simulink model "EjemploClienteConNovint"  (Simulink 7.8)
settings: Solver=ode3  StartTime=0.0  StopTime=inf  FixedStep=0.001  RelTol=1e-3
libraries: aerolibanimutils x1
settings Model: Creator=Usuario  LastModifiedBy=Sebastián
settings OptimizationCC: SimCompilerOptimization=On
settings DebuggingCC: FcnCallInpInsideContextMsg=Use local settings

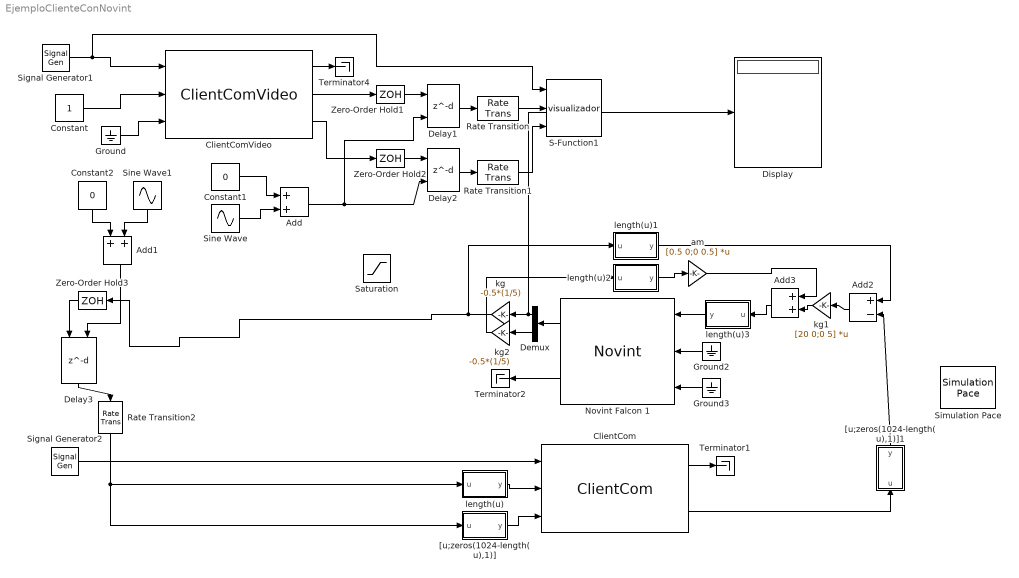
== system EjemploClienteConNovint ==
  Add : Sum  SampleTime=0.05
  Add1 : Sum  SampleTime=0.05
  Add2 : Sum  Inputs=+-
  Add3 : Sum
  ClientCom : S-Function  FunctionName=ClientCom  EnableBusSupport=off
      mask Display:
      | patch([0 4. 4 0],[0.02 0.02 0.98 0.98],0.9*[123 193 255]/255)
      | patch([0 4 4 0],[0.1 0.1 0.9 0.9],[123 193 255]/255)
      | patch([1.5 2.5 2.5 2.3 2.3 1.7 1.7 1.5],[0 0 1 1 1.2 1.2 1 1],[130 130 130]/255)
      | patch([1.3 2.7 2.7 1.3],[1.2 1.2 2.9 2.9],0.85*[130 130 130]/255)
      | patch([1.4 2.6 2.6 1.4],[1.3 1.3 2.8 2.8],[123 193 255]/255)
      | patch([1.5 2.5 2.5 1.5],[1.4 1.4 2.7 2.7],0.85*[130 130 130]/255)
      | patch([1.9 2.1 2.1 1.9],[1.8 1.8 2.1 2.1],[123 193 255]/255)
      | color('red')
      | port_label('input',1,'clock')
      | port_label('input',2,'sizeSend')
      | port_label('input',3,'dataSend')
      | port_label('output',1,'stateChannel')
      | port_label('output',2,'dataRecv')
  ClientComVideo : S-Function  FunctionName=ClientComVideo  EnableBusSupport=off
      mask Display:
      | patch([0 4. 4 0],[0.02 0.02 0.98 0.98],0.9*[123 193 255]/255)
      | patch([0 4 4 0],[0.1 0.1 0.9 0.9],[123 193 255]/255)
      | patch([1.5 2.5 2.5 2.3 2.3 1.7 1.7 1.5],[0 0 1 1 1.2 1.2 1 1],[130 130 130]/255)
      | patch([1.3 2.7 2.7 1.3],[1.2 1.2 2.9 2.9],0.85*[130 130 130]/255)
      | patch([1.4 2.6 2.6 1.4],[1.3 1.3 2.8 2.8],[123 193 255]/255)
      | patch([1.5 2.5 2.5 1.5],[1.4 1.4 2.7 2.7],0.85*[130 130 130]/255)
      | patch([1.9 2.1 2.1 1.9],[1.8 1.8 2.1 2.1],[123 193 255]/255)
      | color('red')
      | port_label('input',1,'clock')
      | port_label('input',2,'sizeSend')
      | port_label('input',3,'dataSend')
      | port_label('output',1,'stateChannel')
      | port_label('output',2,'sizeMustBeRecv')
      | port_label('output',3,'dataRecv')
  Constant : Constant  OutDataTypeStr=uint32
  Constant1 : Constant  Value=0  SampleTime=0.05
  Constant2 : Constant  Value=0  SampleTime=0.05
  Delay1 : Delay  DelayLengthSource=Input port  SampleTime=0.05
      settings: InputPortMap=u0,p1
  Delay2 : Delay  DelayLengthSource=Input port  SampleTime=0.05
      settings: InputPortMap=u0,p1
  Delay3 : Delay  DelayLengthSource=Input port  SampleTime=0.05
      settings: InputPortMap=u0,p1
  Demux : Demux  Outputs=[3 3]
  Display : Display
  Ground : Ground
  Ground2 : Ground
  Ground3 : Ground
  Novint Falcon 1 : S-Function  FunctionName=Novint  Parameters=1  EnableBusSupport=off
      mask Display:
      | color('red')
      | port_label('input',1,'acciones')
      | port_label('input',2,'parametros')
      | port_label('input',3,'parametrosSend')
      | color('blue')
      | port_label('output',1,'estado')
      | port_label('output',2,'botones')
  Rate Transition : RateTransition  OutPortSampleTime=0
  Rate Transition1 : RateTransition  OutPortSampleTime=0
  Rate Transition2 : RateTransition  OutPortSampleTime=0
  S-Function1 : S-Function  FunctionName=visualizador  Parameters=1  EnableBusSupport=off
  Saturation : Saturate
  Signal Generator1 : SignalGenerator  WaveForm=square  Frequency=20
  Signal Generator2 : SignalGenerator  WaveForm=square  Frequency=20
  Simulation Pace : aerolibanimutils/Simulation Pace  SimulationPace=1  SleepMode=MATLAB Thread  OutputPaceError=off  SampleTime=-1
      settings: AttributesFormatString=%<SimulationPace> sec/sec
  Sine Wave : Sin  Amplitude=0  Frequency=0.1*2*pi  SampleTime=0.05
  Sine Wave1 : Sin  Amplitude=0  Frequency=0.1*2*pi  SampleTime=0.05
  Terminator1 : Terminator
  Terminator2 : Terminator
  Terminator4 : Terminator
  Zero-Order Hold1 : ZeroOrderHold  SampleTime=0.05
  Zero-Order Hold2 : ZeroOrderHold  SampleTime=0.05
  Zero-Order Hold3 : ZeroOrderHold  SampleTime=0.05
  "[u;zeros(1024-length(u),1)]" : MATLAB Function  TreatAsAtomicUnit=on
  "[u;zeros(1024-length(u),1)]1" : MATLAB Function  TreatAsAtomicUnit=on
  am : Gain  Gain=[0.5 0;0 0.5]  Multiplication=Matrix(K*u)
  kg : Gain  Gain=-0.5*(1/5)
  kg1 : Gain  Gain=[20 0;0 5]  Multiplication=Matrix(K*u)
  kg2 : Gain  Gain=-0.5*(1/5)
  length(u) : MATLAB Function  TreatAsAtomicUnit=on
  length(u)1 : MATLAB Function  TreatAsAtomicUnit=on
  length(u)2 : MATLAB Function  TreatAsAtomicUnit=on
  length(u)3 : MATLAB Function  TreatAsAtomicUnit=on
  wires:
  ClientComVideo/2 -> Zero-Order Hold1/1
  ClientComVideo/3 -> Zero-Order Hold2/1
  Signal Generator1/1 -> ClientComVideo/1, S-Function1/1
  Constant/1 -> ClientComVideo/2
  Signal Generator2/1 -> ClientCom/1
  length(u)/1(y) -> ClientCom/2
  Novint Falcon 1/1 -> Demux/1
  "[u;zeros(1024-length(u),1)]"/1(y) -> ClientCom/3
  Novint Falcon 1/2 -> Terminator2/1
  ClientCom/1 -> Terminator1/1
  ClientCom/2 -> "[u;zeros(1024-length(u),1)]1"/1(u)
  Ground/1 -> ClientComVideo/3
  ClientComVideo/1 -> Terminator4/1
  Demux/2 -> kg2/1
  Add3/1 -> length(u)3/1(u)
  Ground2/1 -> Novint Falcon 1/2
  Ground3/1 -> Novint Falcon 1/3
  Sine Wave/1 -> Add/2
  Constant1/1 -> Add/1
  Zero-Order Hold1/1 -> Delay1/1
  Zero-Order Hold2/1 -> Delay2/1
  Delay1/1 -> Rate Transition/1
  Delay2/1 -> Rate Transition1/1
  Add/1 -> Delay1/2, Delay2/2
  Rate Transition/1 -> S-Function1/2
  Rate Transition1/1 -> S-Function1/3
  Constant2/1 -> Add1/1
  Delay3/1 -> Rate Transition2/1
  Sine Wave1/1 -> Add1/2
  Rate Transition2/1 -> length(u)/1(u), "[u;zeros(1024-length(u),1)]"/1(u)
  Demux/1 -> kg/1, Display/1
  Add1/1 -> Delay3/2
  length(u)1/1(y) -> Add2/1
  "[u;zeros(1024-length(u),1)]1"/1(y) -> Add2/2
  kg/1 -> Zero-Order Hold3/1, length(u)1/1(u)
  Add2/1 -> kg1/1
  kg2/1 -> length(u)2/1(u)
  length(u)2/1(y) -> am/1
  kg1/1 -> Add3/2
  am/1 -> Add3/1
  length(u)3/1(y) -> Novint Falcon 1/1
  Zero-Order Hold3/1 -> Delay3/1

== matlab function length(u) ==
  data: u input double; y output double
function y = fcn(u)
%#codegen

y = uint32(length(u));

== matlab function [u;zeros(1024-length(u),1)] ==
  data: u input double; y output double
function y = fcn(u)
%#codegen

y = [u;zeros(1024-length(u),1)];

== matlab function [u;zeros(1024-length(u),1)]1 ==
  data: u input double; y output double
function y = fcn(u)
%#codegen

y = [u(4);u(5)];

== matlab function length(u)1 ==
  data: u input double; y output double
function y = fcn(u)
%#codegen

y = [u(3);u(1)];

== matlab function length(u)2 ==
  data: u input double; y output double
function y = fcn(u)
%#codegen

y = [u(3);u(1)];

== matlab function length(u)3 ==
  data: u input double; y output double
function y = fcn(u)
%#codegen

y = [u(2);0;u(1)];
